simulink model "sldemo_tc"  (Simulink 7.6)
settings: Solver=ode3  SolverMode=SingleTasking  StartTime=0.0  StopTime=10.0  FixedStep=0.005  RelTol=1e-3
model workspace (MAT data in the model file):
  e_vs_counts = [-0.236 -0.231386474609 -0.226772949219 -0.222159423828 -0.217545898437 -0.212932373047 -0.208318847656 -0.203705322266 -0.199091796875 -0.194478271484 -0.189864746094 -0.185251220703 ... (4096 elements, 4096x1)]
  TypeS_tdegc_vs_bits = [-50 -48.8466186523 -47.6932373047 -46.6318855286 -45.6364746094 -44.4830932617 -43.3297119141 -42.1763305664 -41.0229492188 -40.0956535339 -38.9661865234 -37.8502426147 ... (4096 elements, 4096x1)]
  TypeS_bits_bp = [0; 50; 100; 150; 200; 250; 300; 350; 400; 450; 500; 550; 600; 650; 700; 750; 800; 850; 900; 950; 1000; 1050; 1100; 1150; 1200; 1250; 1300; 1350; 1400; 1450; 1500; 1550; 1600; 1650; 1700; 1750; 1800; 1850; 1900; 1950; 2000; 2050; 2100; 2150; 2200; 2250; 2300; 2350; 2400; 2450; 2500; 2550; 2600; 2650; 2700; 2750; 2800; 2850; 2900; 2950; 3000; 3050; 3100; 3150; 3200; 3250; 3300; 3350; 3400; 3450; 3500; 3550; 3600; 3650; 3700; 3750; 3800; 3850; 3900; 3950; 4000; 4050; 4095]
  TypeS_tdegc_interp = [-50; -1.05395507812; 38.4789352417; 73.4326858521; 105.529296875; 135.797668457; 164.757202148; 192.63710022; 219.712234497; 246.231826782; 272.095336914; 297.6043396; 322.790588379; 347.53237915; 372.051971436; 396.31439209; 420.382019043; 444.149658203; 467.81729126; 491.284912109; 514.55255127; 537.620178223; 560.587768555; 583.355407715; 606.023071289; 628.490661621; 650.858276367; 673.02355957; 694.994140625; 716.873779297; 738.62878418; 760.178588867; 781.60369873; 802.846984863; 823.999389648; 844.969970703; 865.849609375; 886.547424316; 907.15435791; 927.614562988; 948.004211426; 968.227233887; 988.309387207; 1008.27996826; 1028.22961426; 1047.95263672; 1067.67565918; 1087.23205566; 1106.76916504; 1126.17810059; 1145.56774902; 1164.79077148; 1184.09716797; 1203.23681641; 1222.37658691; 1241.51623535; 1260.57263184; 1279.62890625; 1298.68530273; 1317.74169922; 1336.71472168; 1355.71166992; 1374.74401855; 1393.71704102; 1412.7734375; 1431.82983398; 1450.8861084; 1469.94250488; 1489.08215332; 1508.22192383; 1527.44494629; 1546.66796875; 1565.97424316; 1585.36401367; 1604.83703613; 1624.33825684; 1643.94970703; 1663.67272949; 1683.47912598; 1703.49316406; 1723.91833496; 1744.9777832; 1764.53869629]
  TypeS_T_degC = [-50 -49 -48 -47 -46 -45 -44 -43 -42 -41 -40 -39 ... (1816 elements, 1816x1)]
  TypeS_E_Volts = [-0.000236 -0.000232 -0.000228 -0.000224 -0.000219 -0.000215 -0.000211 -0.000207 -0.000203 -0.000199 -0.000194 -0.00019 ... (1816 elements, 1816x1)]
StartFcn:
  | set_param('sldemo_tc/Scope','Open','on')
values from neighbouring files (symbols this model uses):
  TypeS_bits_bp = single(TypeS_bits_bp)    [sldemo_create_tc_tabledata.m]
  TypeS_tdegc_vs_bits = single(interp1(es,ts,e_vs_counts, 'linear','extrap'))    [sldemo_create_tc_tabledata.m]
libraries: simulink x3, simulink_extras x1
Description:
  | Thermocouple Modeling and Signal Conversion
  | 
  | The thermocouple is one of the popular analog transducers today, along
  | with other devices such as position sensors, strain gages, pressure
  | transducers, and resistance temperature devices (RTDs). Operating under
  | the principle of the Seebeck (or thermoelectric) effect, thermocouples
  | have an empirically determined nonlinear behavior that is well known over
  | each junction type's useful operating range. If you run the model, you
  | will be able to see the cumulative effect of each component on dynamic
  | measurement accuracy. This demonstration will focus on models for each of
  | these components in a dynamic temperature measurement system for a Type S
  | (Platinum-10% Rhodium(+) versus Platinum(-) ) : a thermocouple device and
  | probe assembly, a signal conditioning method, an analog to digital
  | converter (ADC), and a software specification for converting the ADC
  | output back into a temperature value. An additional section shows how to
  | obtain and use standard NIST ITS-90 thermocouple data with Simulink
  | models. Look-up tables and a polynomial block are used in this design to
  | capture the nonlinear behavior of the thermocouple. Note that the
  | polynomial block is a viable alternative to look-up tables for some
  | applications, minimizing ROM usage at the cost of some additional
  | computation for the full polynomial representation.
settings Model: Creator=The MathWorks Inc.  ExtModeAutoUpdateStatusClock=off
settings DataIOCC: SaveOutput=off  SaveTime=off
settings OptimizationCC: InlineParams=on  InlineInvariantSignals=on  InitFltsAndDblsToZero=on  BufferReusableBoundary=off
settings DebuggingCC: SaveWithParameterizedLinksMsg=none  CheckExecutionContextPreStartOutputMsg=on  CheckExecutionContextRuntimeOutputMsg=on  SignalResolutionControl=TryResolveAllWithWarning  MultiTaskDSMMsg=warning  MultiTaskCondExecSysMsg=none  BusObjectLabelMismatch=none
settings HardwareCC: ProdIntDivRoundTo=Floor  ProdEndianess=LittleEndian  ProdHWDeviceType=32-bit xPC Target (AMD Athlon)
settings RTWCC: GenCodeOnly=on  IncludeERTFirstTime=on
settings CodeAppCC: CustomSymbolStrFcn=$F$N$M
settings GRTTargetCC: TargetFcnLib=iso_tfl_tmw.mat  TargetFunctionLibrary=ISO_C

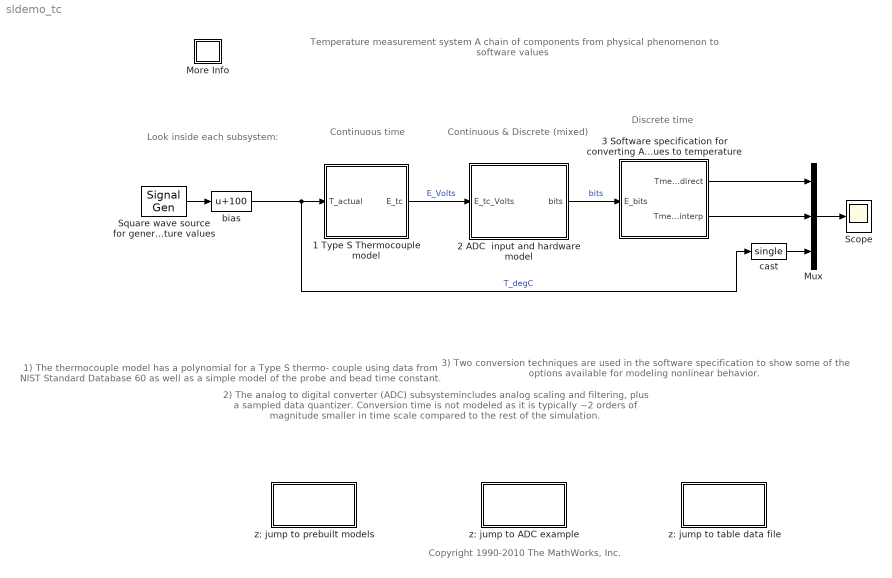
== system sldemo_tc ==
  note: Temperature measurement system
      | A chain of components from
      | physical phenomenon to software values
  note: 1) The thermocouple model has
      | a polynomial for a Type S thermo-
      | couple using data from NIST
      | Standard Database 60 as well
      | as a simple model of the probe
      | and bead time constant.
  note: 2) The analog to digital converter
      | (ADC) subsystemincludes analog
      | scaling and filtering, plus a
      | sampled data quantizer.
      | Conversion time is not modeled
      | as it is typically ~2 orders of
      | magnitude smaller in time scale
      | compared to the rest of the
      | simulation.
  note: 3) Two conversion techniques
      | are used  in the software
      | specification to show some
      | of the options available for
      | modeling nonlinear behavior.
  note: Continuous
      | time
  note: Discrete
      | time
  note: Continuous &
      | Discrete (mixed)
  note: Look inside
      | each subsystem:
  note: Copyright 1990-2010 The MathWorks, Inc.
  1 Type S Thermocouple model : Subsystem
  2 ADC  input and hardware model : Subsystem
  3 Software specification for converting ADC values to temperature : Subsystem
  More Info : Subsystem
      settings: OpenFcn=showdemo('sldemo_tc_script')
      mask Display: disp('?')
  Mux : Mux  Inputs=3
  Scope : Scope
      settings: TimeRange=10  YMin=-25  YMax=225
  Square wave source for generating temperature values : SignalGenerator  WaveForm=square  Amplitude=100
  bias : Bias  Bias=100
  cast : DataTypeConversion  OutDataTypeStr=single
  z: jump to ADC example : Subsystem
      settings: OpenFcn=open_system('sldemo_adc_quantize','force')
      mask Type: ADC quantizer details
      mask Description: Jump to a model that exercises more details of the behavior of the Idealized ADC quantizer block that is part of the hardware model.
      mask Display: disp('ADC Quantizer\nDetails')
  z: jump to prebuilt models : Subsystem
      settings: OpenFcn=open_system('sldemo_tc_blocks','force')
      mask Type: ADC quantizer details
      mask Description: Jump to a model that exercises more details of the behavior of the Idealized ADC quantizer block that is part of the hardware model.
      mask Display: disp('Additional\nThermocouple\nModels')
  z: jump to table data file : Subsystem
      settings: OpenFcn=edit sldemo_create_tc_tabledata.m
      mask Type: ADC quantizer details
      mask Description: Jump to a model that exercises more details of the behavior of the Idealized ADC quantizer block that is part of the hardware model.
      mask Display: disp('Table Design\nDetails')
  wires:
  3 Software specification for converting ADC values to temperature/1(Tmeas_direct) -> Mux/1
  1 Type S Thermocouple model/1(E_tc) -> 2 ADC  input and hardware model/1(E_tc_Volts)  "E_Volts"
  2 ADC  input and hardware model/1(bits) -> 3 Software specification for converting ADC values to temperature/1(E_bits)  "bits"
  3 Software specification for converting ADC values to temperature/2(Tmeas_interp) -> Mux/2
  Mux/1 -> Scope/1
  bias/1 -> 1 Type S Thermocouple model/1(T_actual), cast/1  "T_degC"
  Square wave source for generating temperature values/1 -> bias/1
  cast/1 -> Mux/3

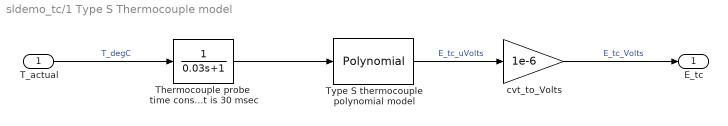
== system sldemo_tc/1 Type S Thermocouple model ==
  T_actual : Inport
  Thermocouple probe  time constant is 30 msec : TransferFcn  Denominator=[0.03 1]
  Type S thermocouple polynomial model : simulink/Math Operations/Polynomial  Description=|  coefs=[ +2.71443176145e-021, -1.25068871393e-017, +2.55744251786e-014, -3.31465196389e-011, +3.22028823036e-008, -2.32477968689e-005, +1.25934289740e-002, +5.40313308631e+000, +0.00000000000e+000 ]
      | 0 deg C ice reference         
      |       microVolts = f(Temperature degC)   
      | (Segment 1) input range: -50 to 1063 degC
      settings: AttributesFormatString=%<Description>
  cvt_to_Volts : Gain  Gain=1e-6
  E_tc : Outport
  wires:
  Thermocouple probe  time constant is 30 msec/1 -> Type S thermocouple polynomial model/1
  T_actual/1 -> Thermocouple probe  time constant is 30 msec/1  "T_degC"
  Type S thermocouple polynomial model/1 -> cvt_to_Volts/1  "E_tc_uVolts"
  cvt_to_Volts/1 -> E_tc/1  "E_tc_Volts"

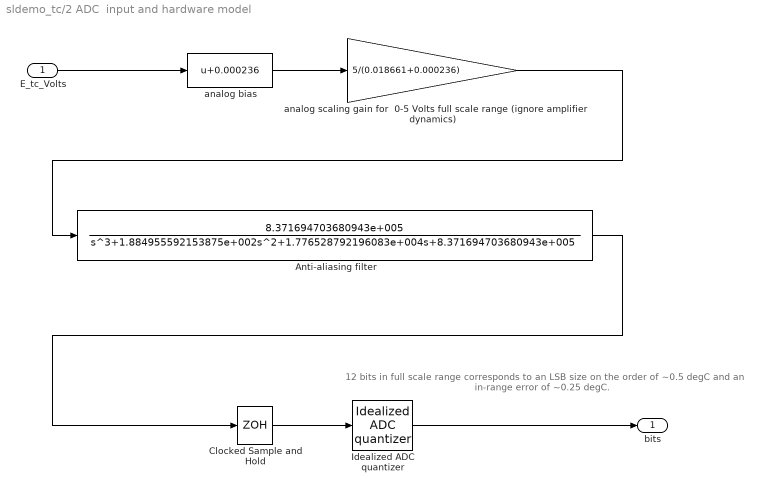
== system sldemo_tc/2 ADC  input and hardware model ==
  note: 12 bits in full scale range corresponds to
      | an LSB size on the order of ~0.5 degC and
      | an in-range error of ~0.25 degC.
  E_tc_Volts : Inport
  Anti-aliasing filter : TransferFcn  Description=|  Numerator=8.371694703680943e+005  Denominator=[ 1, 1.884955592153875e+002, 1.776528792196083e+004, 8.371694703680943e+005 ]
      | Designed using Signal Processing Toolbox command:
      | >> [num,den] = butter(3,15*2*pi,'low','s')
      settings: AttributesFormatString=%<Description>
  Clocked Sample and Hold : ZeroOrderHold  SampleTime=0.020
      settings: AttributesFormatString=(%<SampleTime> sec)
  Idealized ADC quantizer : simulink_extras/Additional Discrete/Idealized ADC quantizer  NumberOfConverterBits=12  Vmin=0  Vmax=5  OutputDataType=uint16  OutputNegativeValues=off
  analog bias : Bias  Bias=0.000236
  analog scaling gain for  0-5 Volts full scale range (ignore amplifier dynamics) : Gain  Gain=5/(0.018661+0.000236)
  bits : Outport
  wires:
  analog scaling gain for  0-5 Volts full scale range (ignore amplifier dynamics)/1 -> Anti-aliasing filter/1
  E_tc_Volts/1 -> analog bias/1
  Clocked Sample and Hold/1 -> Idealized ADC quantizer/1
  Idealized ADC quantizer/1 -> bits/1
  analog bias/1 -> analog scaling gain for  0-5 Volts full scale range (ignore amplifier dynamics)/1
  Anti-aliasing filter/1 -> Clocked Sample and Hold/1

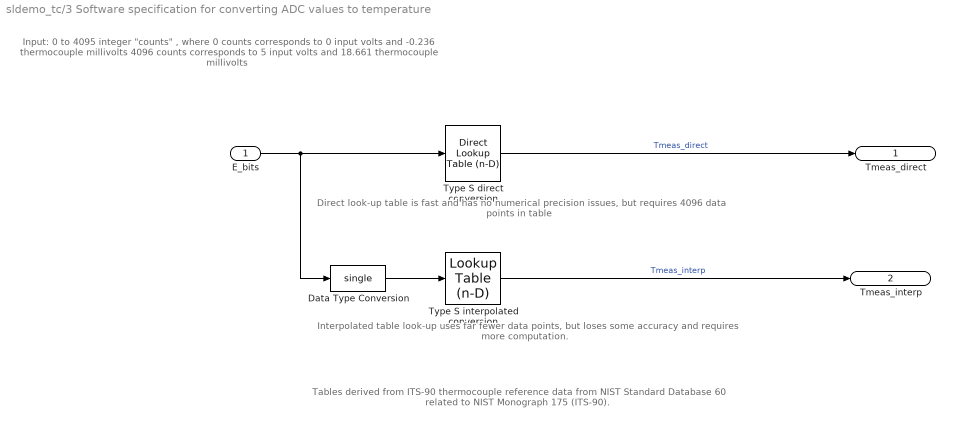
== system sldemo_tc/3 Software specification for converting ADC values to temperature ==
  note: Input: 0 to 4095 integer "counts" , where
      |             0        counts corresponds to 0 input volts and -0.236 thermocouple millivolts
      |             4096 counts corresponds to 5 input volts and 18.661 thermocouple millivolts
  note: Tables derived from ITS-90 thermocouple reference data
      | from NIST Standard Database 60 related to NIST Monograph 175 (ITS-90).
  note: Direct look-up table is fast and has no numerical precision issues,
      | but requires 4096 data points in table
  note: Interpolated table look-up uses far fewer data points,
      | but loses some accuracy and requires more computation.
  E_bits : Inport  OutDataTypeStr=uint16
  Data Type Conversion : DataTypeConversion  OutDataTypeStr=single
  Type S direct conversion : simulink/Lookup Tables/Direct Lookup Table (n-D)  maskTabDims=1  explicitNumDims=1  outDims=Element  tabIsInput=off  mxTable=TypeS_tdegc_vs_bits  clipFlag=Warning
      settings: AttributesFormatString=(%<mxTable>)
  Type S interpolated conversion : simulink/Lookup Tables/Lookup Table (n-D)  numDimsPopupSelect=1  bp1=TypeS_bits_bp  bp2=[10,22,31]  bp3=[1:3]  bp4=[1:3]  bpcell={ [1:3], [1:3] }  explicitNumDims=2  searchMode=Linear Search  cacheBpFlag=on  vectorInputFlag=off  tableData=TypeS_tdegc_interp  interpMethod=Linear  extrapMethod=None - Clip  rangeErrorMode=Warning
      settings: AttributesFormatString=(%<tableData>)
  Tmeas_direct : Outport
  Tmeas_interp : Outport  Port=2
  wires:
  E_bits/1 -> Type S direct conversion/1, Data Type Conversion/1
  Type S direct conversion/1 -> Tmeas_direct/1  "Tmeas_direct"
  Data Type Conversion/1 -> Type S interpolated conversion/1
  Type S interpolated conversion/1 -> Tmeas_interp/1  "Tmeas_interp"

== system sldemo_tc/More Info ==

== system sldemo_tc/z: jump to ADC example ==
  note: This block intentionally has no contents.

== system sldemo_tc/z: jump to prebuilt models ==
  note: This block intentionally has no contents.

== system sldemo_tc/z: jump to table data file ==
  note: This block intentionally has no contents.
